simulink model "nadir_pointing"  (R2021a)
settings: Solver=VariableStepAuto  StartTime=0.0  StopTime=Torb  RelTol=1e-3
values from neighbouring files (symbols this model uses):
  Tmax = Fmax*Larm    (= 0.00125)    [params_nadir.m]
libraries: sharedtransform x2
settings Model: Creator=Laura  LastModifiedBy=Laura

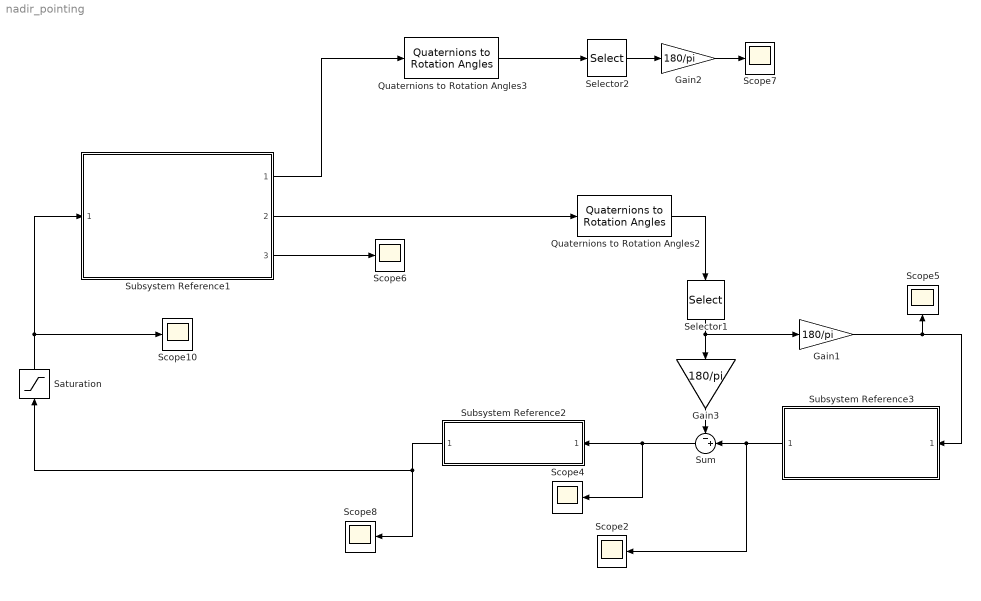
== system nadir_pointing ==
  Gain1 : Gain  Gain=180/pi
  Gain2 : Gain  Gain=180/pi
  Gain3 : Gain  Gain=180/pi
  Quaternions to Rotation Angles2 : sharedtransform/Quaternions to Rotation Angles  rotationOrder=ZYX  aMode=aMode
      settings: SourceProductBaseCode=AE,PW,DR,MT,UV,VE
  Quaternions to Rotation Angles3 : sharedtransform/Quaternions to Rotation Angles  rotationOrder=ZYX  aMode=aMode
      settings: SourceProductBaseCode=AE,PW,DR,MT,UV,VE
  Saturation : Saturate  UpperLimit=Tmax  LowerLimit=-Tmax
  Scope{2,4..8,10} (7 alike) : Scope
  Selector1 : Selector  InputPortWidth=3  IndexOptions=Index vector (dialog)  Indices=[3 2 1]  OutputSizes=1
  Selector2 : Selector  InputPortWidth=3  IndexOptions=Index vector (dialog)  Indices=[3 2 1]  OutputSizes=1
  Subsystem Reference1 : Subsystem  ReferencedSubsystem=DKE_nadirpointing
  Subsystem Reference2 : Subsystem  ReferencedSubsystem=PID
  Subsystem Reference3 : Subsystem  ReferencedSubsystem=ThreeAxesSignals
  Sum : Sum  Inputs=-+|
  wires:
  Quaternions to Rotation Angles2/1 -> Selector1/1
  Selector1/1 -> Gain1/1, Gain3/1
  Sum/1 -> Scope4/1, Subsystem Reference2/1
  Subsystem Reference1/3 -> Scope6/1
  Subsystem Reference1/1 -> Quaternions to Rotation Angles3/1
  Gain1/1 -> Subsystem Reference3/1, Scope5/1
  Quaternions to Rotation Angles3/1 -> Selector2/1
  Selector2/1 -> Gain2/1
  Gain2/1 -> Scope7/1
  Subsystem Reference3/1 -> Scope2/1, Sum/2
  Gain3/1 -> Sum/1
  Subsystem Reference1/2 -> Quaternions to Rotation Angles2/1
  Subsystem Reference2/1 -> Scope8/1, Saturation/1
  Saturation/1 -> Subsystem Reference1/1, Scope10/1
